simulink model "DSB_SCAM"  (R2021a)
settings: Solver=VariableStepAuto  StartTime=0.0  StopTime=10.0  RelTol=1e-3
libraries: commanapbnd3 x3
settings Model: Creator=Arif  LastModifiedBy=Arif

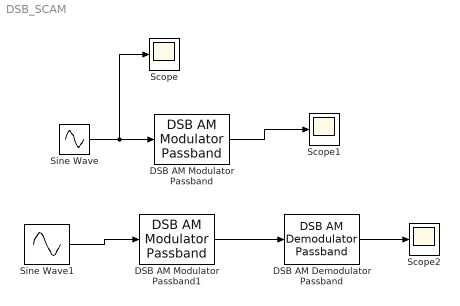
== system DSB_SCAM ==
  DSB AM Demodulator Passband : commanapbnd3/DSB AM Demodulator Passband  Fc=2000  Ph=0  method=Butterworth  n=4  cf=300  Rp=0.1  Rs=50  Offset=1
      settings: SourceProductBaseCode=CM
  DSB AM Modulator Passband : commanapbnd3/DSB AM Modulator Passband  Fc=1500  Ph=0  Offset=1
      settings: SourceProductBaseCode=CM
  DSB AM Modulator Passband1 : commanapbnd3/DSB AM Modulator Passband  Fc=2000  Ph=0  Offset=1
      settings: SourceProductBaseCode=CM
  Scope : Scope
  Scope1 : Scope
  Scope2 : Scope
  Sine Wave : Sin  SineType=Sample based  Samples=800  SampleTime=0.0001
  Sine Wave1 : Sin  SineType=Sample based  Samples=500  SampleTime=0.0001  Offset=500
  wires:
  Sine Wave/1 -> Scope/1, DSB AM Modulator Passband/1
  DSB AM Modulator Passband/1 -> Scope1/1
  Sine Wave1/1 -> DSB AM Modulator Passband1/1
  DSB AM Modulator Passband1/1 -> DSB AM Demodulator Passband/1
  DSB AM Demodulator Passband/1 -> Scope2/1
